simulink model "PIDvsGs"  (R2020b)
settings: Solver=VariableStepAuto  StartTime=0.0  StopTime=10.0  RelTol=1e-3
values from neighbouring files (symbols this model uses):
  g = 9.81    [params.m]
  I = m1*r1^2+m2*r2^2+m3*r3^2    (= 0.0018475)    [params.m]
  m1 = 0.031    [params.m]
  r1 = 0.19    [params.m]
undefined symbols (not defined in the file or in its folder): alfa_r, Fpv, Kc, kf, Td, Ti
settings Model: Creator=bou  LastModifiedBy=bou

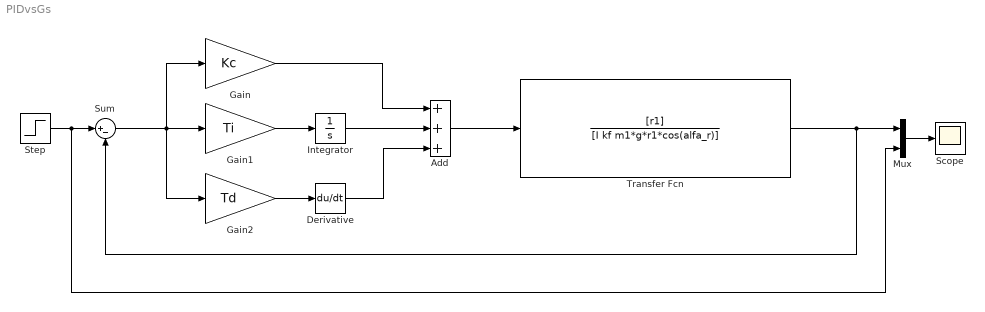
== system PIDvsGs ==
  Add : Sum  Inputs=+++
  Derivative : Derivative
  Gain : Gain  Gain=Kc
  Gain1 : Gain  Gain=Ti
  Gain2 : Gain  Gain=Td
  Integrator : Integrator
  Mux : Mux  Inputs=2
  Scope : Scope
  Step : Step  After=Fpv  SampleTime=0
  Sum : Sum  Inputs=|+-
  Transfer Fcn : TransferFcn  Numerator=[r1]  Denominator=[I kf m1*g*r1*cos(alfa_r)]
  wires:
  Integrator/1 -> Add/2
  Derivative/1 -> Add/3
  Gain/1 -> Add/1
  Gain1/1 -> Integrator/1
  Gain2/1 -> Derivative/1
  Sum/1 -> Gain2/1, Gain/1, Gain1/1
  Add/1 -> Transfer Fcn/1
  Transfer Fcn/1 -> Sum/2, Mux/1
  Step/1 -> Mux/2, Sum/1
  Mux/1 -> Scope/1
